simulink model "Direct_Dynamics6DOF"  (R2018b)
settings: Solver=ode4  StartTime=0.0  StopTime=10  FixedStep=0.05  RelTol=1e-3
settings Model: Creator=root  LastModifiedBy=root

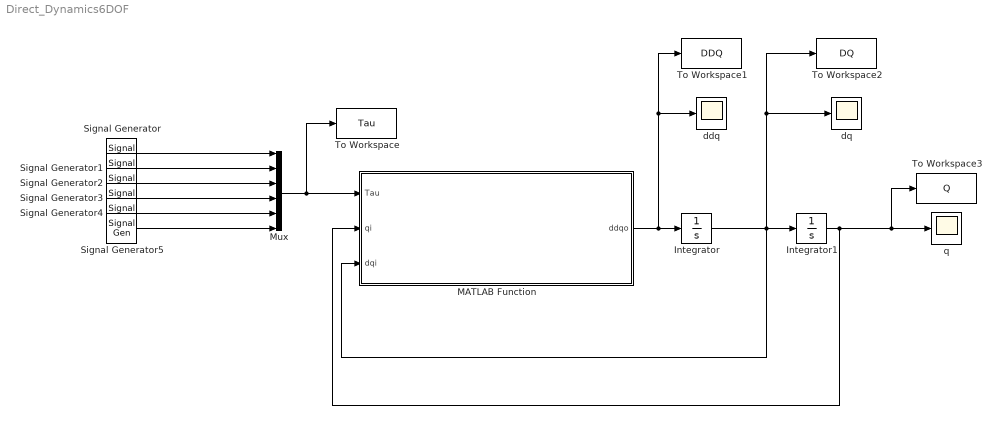
== system Direct_Dynamics6DOF ==
  Integrator : Integrator
  Integrator1 : Integrator
  MATLAB Function : MATLAB Function  TreatAsAtomicUnit=on
  Mux : Mux  Inputs=6
  Signal Generator : SignalGenerator  Frequency=0.5  Units=rad/sec
  Signal Generator1 : SignalGenerator  Frequency=0.4  Units=rad/sec
  Signal Generator2 : SignalGenerator  Frequency=0.3  Units=rad/sec
  Signal Generator3 : SignalGenerator  Frequency=0.2  Units=rad/sec
  Signal Generator4 : SignalGenerator  Frequency=0.1  Units=rad/sec
  Signal Generator5 : SignalGenerator  Frequency=0.6  Units=rad/sec
  To Workspace : ToWorkspace  VariableName=Tau  SampleTime=-1
  To Workspace1 : ToWorkspace  VariableName=DDQ  SampleTime=-1
  To Workspace2 : ToWorkspace  VariableName=DQ  SampleTime=-1
  To Workspace3 : ToWorkspace  VariableName=Q  SampleTime=-1
  ddq : Scope
  dq : Scope
  q : Scope
  wires:
  Integrator/1 -> To Workspace2/1, dq/1, Integrator1/1, MATLAB Function/3(dqi)
  Integrator1/1 -> To Workspace3/1, q/1, MATLAB Function/2(qi)
  Mux/1 -> To Workspace/1, MATLAB Function/1(Tau)
  Signal Generator/1 -> Mux/1
  Signal Generator1/1 -> Mux/2
  Signal Generator2/1 -> Mux/3
  Signal Generator3/1 -> Mux/4
  Signal Generator4/1 -> Mux/5
  Signal Generator5/1 -> Mux/6
  MATLAB Function/1(ddqo) -> To Workspace1/1, ddq/1, Integrator/1

== matlab function Direct_Dynamics6DOF/MATLAB Function ==
  data: Tau input; ddqo output; qi input; dqi input
function ddqo   = DirectDynamics(Tau,qi,dqi)
    ddqo = zeros(1,6);
    coder.extrinsic('SolveSyms');
    c = zeros(6,1);
    m = zeros(6,6);
    g = zeros(6,1);
    [m,c,g] = SolveSyms(qi,dqi);
    ddqo(1:6) = m\((Tau(1:6))-c-g);
end
